simulink model "f8_VPP_demo_DER2"  (R2019b)
settings: Solver=VariableStepAuto  StartTime=0.0  StopTime=2  RelTol=1e-3
PreLoadFcn:
  | sr=0;ss=1;
InitFcn:
  | sr=0;ss=1;
undefined symbols (not defined in the file): Ion, Lithium
libraries: powerlib x185, powerlib_meascontrol x45, electricdrivelib x3, re_lib x3
(part 2 of 2)

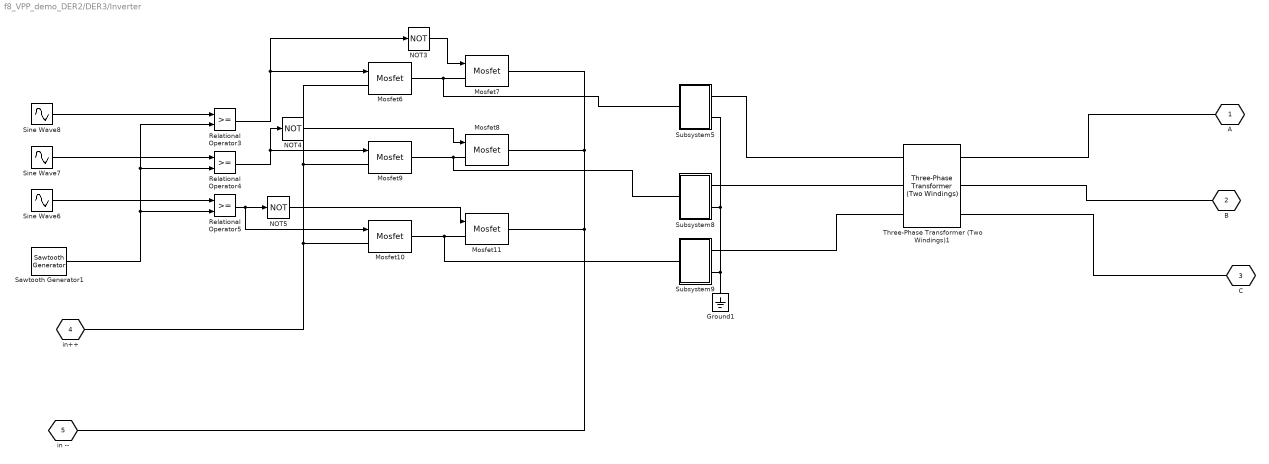
== system f8_VPP_demo_DER2/DER3/Inverter ==
  Ground1 : powerlib/Elements/Ground  LConnTagsString=a
      settings: SourceProductName=Simscape Electrical
  Mosfet{6..11} (6 alike) : powerlib/Power Electronics/Mosfet  Ron=0.1  Lon=0  Rd=0.01  Vfd=0  IC=0  Rs=1e5  Cs=inf  Measurements=off
      settings: SourceProductName=Simscape Electrical
  NOT3 : Logic  Operator=NOT  IconShape=distinctive  AllPortsSameDT=off  OutDataTypeStr=boolean
  NOT4 : Logic  Operator=NOT  IconShape=distinctive  AllPortsSameDT=off  OutDataTypeStr=boolean
  NOT5 : Logic  Operator=NOT  IconShape=distinctive  AllPortsSameDT=off  OutDataTypeStr=boolean
  Relational Operator3 : RelationalOperator  OutDataTypeStr=boolean  ZeroCross=off  RndMeth=Simplest
  Relational Operator4 : RelationalOperator  OutDataTypeStr=boolean  ZeroCross=off  RndMeth=Simplest
  Relational Operator5 : RelationalOperator  OutDataTypeStr=boolean  ZeroCross=off  RndMeth=Simplest
  Sawtooth Generator1 : powerlib_meascontrol/Pulse & Signal Generators/Sawtooth Generator  Freq=1e3  Phase=180  Ts=0
      settings: SourceProductName=Simscape Electrical
  Sine Wave6 : Sin  Frequency=2*pi*50  Phase=4*pi/3  SampleTime=0
  Sine Wave7 : Sin  Frequency=2*pi*50  Phase=2*pi/3  SampleTime=0
  Sine Wave8 : Sin  Frequency=2*pi*50  SampleTime=0
  Subsystem5 : Subsystem
  Subsystem8 : Subsystem
  Subsystem9 : Subsystem
  Three-Phase Transformer (Two Windings)1 : powerlib/Elements/Three-Phase Transformer (Two Windings)  Winding1Connection=Yg  Winding2Connection=Yg  CoreType=Three single-phase transformers  SetSaturation=off  Hysteresis=off  DataFile='hysteresis'  SetInitialFlux=off  Measurements=None  UNITS=pu  NominalPower=[ 1e3 , 50 ]  Winding1=[ 31.5 , 0.002 , 0.08 ]  Winding2=[ 240 , 0.002 , 0.08 ]  Rm=500  Lm=500  L0=0.5  Saturation=[ 0,0 ; 0.0024,1.2 ; 1.0,1.52 ]  InitialFluxes=[ 0.8 , -0.8 , 0.7 ]  BreakLoop=off  DiscreteSolver=Trapezoidal iterative  DataType=off  TransfoNumber=1
      settings: SourceProductName=Simscape Electrical
  A : PMIOPort  Tag=PMCPort  Side=Right
  B : PMIOPort  Tag=PMCPort  Port=2  Side=Right
  C : PMIOPort  Tag=PMCPort  Port=3  Side=Right
  in++ : PMIOPort  Tag=PMCPort  Port=4  Side=Left
  in -- : PMIOPort  Tag=PMCPort  Port=5  Side=Left
  wires:
  NOT5/1 -> Mosfet11/1
  Sine Wave6/1 -> Relational Operator5/1
  Sine Wave7/1 -> Relational Operator4/1
  Relational Operator4/1 -> Mosfet9/1, NOT4/1
  NOT4/1 -> Mosfet8/1
  Sawtooth Generator1/1 -> Relational Operator3/2, Relational Operator4/2, Relational Operator5/2
  Sine Wave8/1 -> Relational Operator3/1
  NOT3/1 -> Mosfet7/1
  Relational Operator5/1 -> Mosfet10/1, NOT5/1
  Relational Operator3/1 -> NOT3/1, Mosfet6/1
  connections:
  Mosfet10/LConn1 -- in++/RConn1 -- Mosfet9/LConn1 -- Mosfet6/LConn1
  Three-Phase Transformer (Two Windings)1/LConn3 -- Subsystem9/RConn1
  Mosfet9/RConn1 -- Mosfet8/LConn1 -- Subsystem8/LConn1
  Subsystem8/RConn1 -- Three-Phase Transformer (Two Windings)1/LConn2
  Mosfet11/LConn1 -- Mosfet10/RConn1 -- Subsystem9/LConn1
  Three-Phase Transformer (Two Windings)1/LConn1 -- Subsystem5/RConn1
  Mosfet6/RConn1 -- Mosfet7/LConn1 -- Subsystem5/LConn1
  Mosfet7/RConn1 -- Mosfet8/RConn1 -- in --/RConn1 -- Mosfet11/RConn1
  Subsystem9/RConn2 -- Ground1/LConn1 -- Subsystem8/RConn2 -- Subsystem5/RConn2
  Three-Phase Transformer (Two Windings)1/RConn3 -- C/RConn1
  Three-Phase Transformer (Two Windings)1/RConn2 -- B/RConn1
  Three-Phase Transformer (Two Windings)1/RConn1 -- A/RConn1

== system f8_VPP_demo_DER2/DER3/breaker_3phase1 ==
  c_breaker : Inport
  Breaker : powerlib/Elements/Breaker  InitialState=0  SwitchingTimes="[1/60  5/60]"  External=on  BreakerResistance=0.01  SnubberResistance=1e6  SnubberCapacitance=inf  Measurements=None  MoreParameters=on  NoBreakLoop=off
      settings: SourceProductName=Simscape Electrical
  Breaker1 : powerlib/Elements/Breaker  InitialState=0  SwitchingTimes="[1/60  5/60]"  External=on  BreakerResistance=0.01  SnubberResistance=1e6  SnubberCapacitance=inf  Measurements=None  MoreParameters=on  NoBreakLoop=off
      settings: SourceProductName=Simscape Electrical
  Breaker2 : powerlib/Elements/Breaker  InitialState=0  SwitchingTimes="[1/60  5/60]"  External=on  BreakerResistance=0.01  SnubberResistance=1e6  SnubberCapacitance=inf  Measurements=None  MoreParameters=on  NoBreakLoop=off
      settings: SourceProductName=Simscape Electrical
  a : PMIOPort  Tag=PMCPort  Side=Right
  A : PMIOPort  Tag=PMCPort  Port=2  Side=Left
  B : PMIOPort  Tag=PMCPort  Port=3  Side=Left
  C : PMIOPort  Tag=PMCPort  Port=4  Side=Left
  b : PMIOPort  Tag=PMCPort  Port=5  Side=Right
  c : PMIOPort  Tag=PMCPort  Port=6  Side=Right
  wires:
  c_breaker/1 -> Breaker1/1, Breaker2/1, Breaker/1
  connections:
  B/RConn1 -- Breaker1/LConn1
  A/RConn1 -- Breaker/LConn1
  c/RConn1 -- Breaker2/RConn1
  a/RConn1 -- Breaker/RConn1
  b/RConn1 -- Breaker1/RConn1
  C/RConn1 -- Breaker2/LConn1

== system f8_VPP_demo_DER2/DER3/power Measurement ==
  Current Measurement1 : powerlib/Measurements/Current Measurement  PhasorSimulation=off  OutputType=Complex  PSBequivalent=0
      settings: SourceProductName=Simscape Electrical
  First-Order Filter : powerlib_meascontrol/Filters/First-Order Filter  FilterType=Lowpass  Tc=100e-3  Ts=0  Initialize=off  Vac_Init=[0, 0, 50]  Vdc_Init=0  PlotResponse=off  FreqRange="[0,  200,  1]"
      settings: SourceProductName=Simscape Electrical
  First-Order Filter1 : powerlib_meascontrol/Filters/First-Order Filter  FilterType=Lowpass  Tc=100e-3  Ts=0  Initialize=off  Vac_Init=[0, 0, 50]  Vdc_Init=0  PlotResponse=off  FreqRange="[0,  200,  1]"
      settings: SourceProductName=Simscape Electrical
  Gain : Gain  Gain=3
  Ground1 : powerlib/Elements/Ground  LConnTagsString=a
      settings: SourceProductName=Simscape Electrical
  Product : Product
  RMS : powerlib_meascontrol/Measurements/RMS  TrueRMS=on  Freq=50  RMSInit=210  Ts=0.001
      settings: SourceProductName=Simscape Electrical
  RMS1 : powerlib_meascontrol/Measurements/RMS  TrueRMS=on  Freq=50  RMSInit=210  Ts=0.001
      settings: SourceProductName=Simscape Electrical
  Scope{,1..3} (4 alike) : Scope
  Voltage Measurement1 : powerlib/Measurements/Voltage Measurement  PhasorSimulation=off  OutputType=Complex  PSBequivalent=0
      settings: SourceProductName=Simscape Electrical
  "out " : PMIOPort  Tag=PMCPort  Side=Right
  in : PMIOPort  Tag=PMCPort  Port=2  Side=Left
  m : Outport
  wires:
  Current Measurement1/1 -> Scope1/1, RMS1/1
  Gain/1 -> m/1
  RMS/1 -> First-Order Filter/1
  RMS1/1 -> First-Order Filter1/1
  Voltage Measurement1/1 -> Scope/1, RMS/1
  First-Order Filter1/1 -> Product/1, Scope2/1
  First-Order Filter/1 -> Scope3/1, Product/2
  Product/1 -> Gain/1
  connections:
  Ground1/LConn1 -- Voltage Measurement1/LConn2
  Current Measurement1/LConn1 -- in/RConn1 -- Voltage Measurement1/LConn1
  "out "/RConn1 -- Current Measurement1/RConn1

== system f8_VPP_demo_DER2/DER3/solar system  ==
  Temp : Inport
  Irr : Inport  Port=2
  Bus Selector : BusSelector  OutputSignals=V_PV
  Current Measurement1 : powerlib/Measurements/Current Measurement  PhasorSimulation=off  OutputType=Complex  PSBequivalent=0
  PV Array : re_lib/Solar/PV Array  Npar=40  Nser=10  PlotType=array @ 1000 W/m2 & specified temperatures  S_vec="[ 1000  500  100 ]"  Temp_C_vec="[ 45 25  ]"  ModuleName=1Soltech 1STH-215-P  PlotWhenSelected=off  Pm=213.15  Ncell=60  Voc=36.3  Isc=7.84  Vm=29  Im=7.35  beta_Voc_pc=-0.36099  alpha_Isc_pc=0.102  beta_Voc=-0.13104  alpha_Isc=0.007997  IL=7.8649  I0=2.9259e-10  nI=0.98117  Rsh=313.3991  Rs=0.39383  BAL=off  Tc=1e-6  Tfilter=5e-5
      settings: SourceProductName=Simscape Electrical
  Scope2 : Scope
  Scope3 : Scope
  Series RLC Branch1 : powerlib/Elements/Series RLC Branch  LConnTagsString=__new0  RConnTagsString=__new0  BranchType=R  Resistance=1000000  Inductance=1e-3  SetiL0=off  InitialCurrent=0  Capacitance=1e-6  Setx0=off  InitialVoltage=0  Measurements=None
      settings: SourceProductName=Simscape Electrical
  baterry ++ : PMIOPort  Tag=PMCPort  Side=Right
  baterry -- : PMIOPort  Tag=PMCPort  Port=2  Side=Right
  wires:
  Current Measurement1/1 -> Scope3/1
  Temp/1 -> PV Array/2
  Irr/1 -> PV Array/1
  PV Array/1 -> Bus Selector/1
  Bus Selector/1 -> Scope2/1  "<V_PV>"
  connections:
  PV Array/RConn2 -- baterry --/RConn1 -- Series RLC Branch1/RConn1
  Current Measurement1/RConn1 -- baterry ++/RConn1
  PV Array/RConn1 -- Current Measurement1/LConn1 -- Series RLC Branch1/LConn1

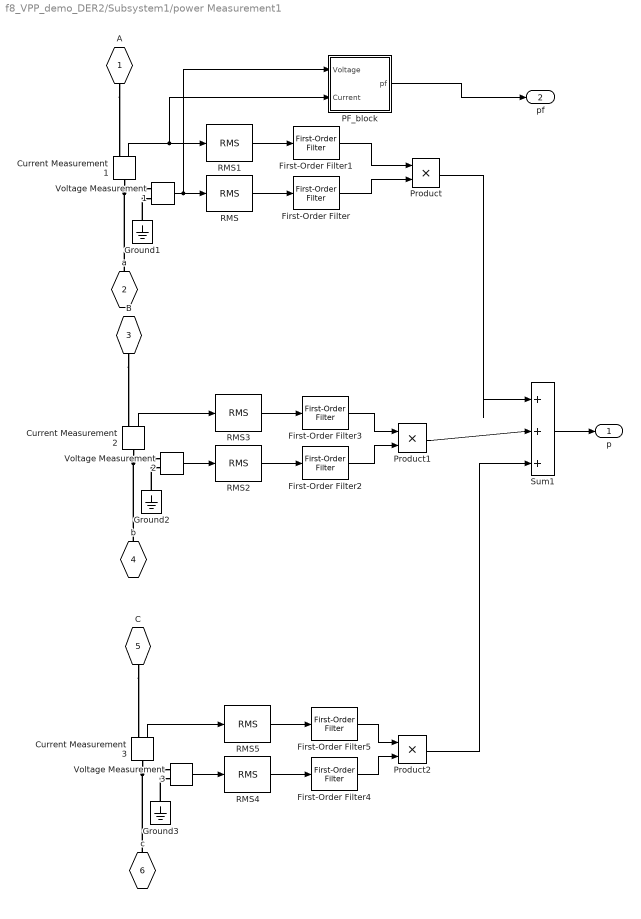
== system f8_VPP_demo_DER2/Subsystem1/power Measurement1 ==
  Current Measurement1 : powerlib/Measurements/Current Measurement  PhasorSimulation=off  OutputType=Complex  PSBequivalent=0
      settings: SourceProductName=Simscape Electrical
  Current Measurement2 : powerlib/Measurements/Current Measurement  PhasorSimulation=off  OutputType=Complex  PSBequivalent=0
      settings: SourceProductName=Simscape Electrical
  Current Measurement3 : powerlib/Measurements/Current Measurement  PhasorSimulation=off  OutputType=Complex  PSBequivalent=0
      settings: SourceProductName=Simscape Electrical
  First-Order Filter{,1..5} (6 alike) : powerlib_meascontrol/Filters/First-Order Filter  FilterType=Lowpass  Tc=100e-3  Ts=0  Initialize=off  Vac_Init=[0, 0, 50]  Vdc_Init=0  PlotResponse=off  FreqRange="[0,  200,  1]"
      settings: SourceProductName=Simscape Electrical
  Ground1 : powerlib/Elements/Ground  LConnTagsString=a
      settings: SourceProductName=Simscape Electrical
  Ground2 : powerlib/Elements/Ground  LConnTagsString=a
      settings: SourceProductName=Simscape Electrical
  Ground3 : powerlib/Elements/Ground  LConnTagsString=a
      settings: SourceProductName=Simscape Electrical
  PF_block : Subsystem
  Product : Product
  Product1 : Product
  Product2 : Product
  RMS{,1..5} (6 alike) : powerlib_meascontrol/Measurements/RMS  TrueRMS=on  Freq=50  RMSInit=210  Ts=0.001
      settings: SourceProductName=Simscape Electrical
  Sum1 : Sum  Inputs=|+++
  Voltage Measurement1 : powerlib/Measurements/Voltage Measurement  PhasorSimulation=off  OutputType=Complex  PSBequivalent=0
      settings: SourceProductName=Simscape Electrical
  Voltage Measurement2 : powerlib/Measurements/Voltage Measurement  PhasorSimulation=off  OutputType=Complex  PSBequivalent=0
      settings: SourceProductName=Simscape Electrical
  Voltage Measurement3 : powerlib/Measurements/Voltage Measurement  PhasorSimulation=off  OutputType=Complex  PSBequivalent=0
      settings: SourceProductName=Simscape Electrical
  "A " : PMIOPort  Tag=PMCPort  Side=Right
  a : PMIOPort  Tag=PMCPort  Port=2  Side=Left
  B : PMIOPort  Tag=PMCPort  Port=3  Side=Right
  b : PMIOPort  Tag=PMCPort  Port=4  Side=Left
  C : PMIOPort  Tag=PMCPort  Port=5  Side=Right
  c : PMIOPort  Tag=PMCPort  Port=6  Side=Left
  p : Outport
  pf : Outport  Port=2
  wires:
  Current Measurement1/1 -> PF_block/2(Current), RMS1/1
  Sum1/1 -> p/1
  RMS/1 -> First-Order Filter/1
  RMS1/1 -> First-Order Filter1/1
  Voltage Measurement1/1 -> PF_block/1(Voltage), RMS/1
  First-Order Filter1/1 -> Product/1
  First-Order Filter/1 -> Product/2
  Product/1 -> Sum1/1
  Voltage Measurement2/1 -> RMS2/1
  RMS3/1 -> First-Order Filter3/1
  RMS2/1 -> First-Order Filter2/1
  Current Measurement2/1 -> RMS3/1
  Current Measurement3/1 -> RMS5/1
  RMS4/1 -> First-Order Filter4/1
  RMS5/1 -> First-Order Filter5/1
  Voltage Measurement3/1 -> RMS4/1
  First-Order Filter3/1 -> Product1/1
  First-Order Filter2/1 -> Product1/2
  First-Order Filter5/1 -> Product2/1
  First-Order Filter4/1 -> Product2/2
  Product1/1 -> Sum1/2
  Product2/1 -> Sum1/3
  PF_block/1(pf) -> pf/1
  connections:
  Ground1/LConn1 -- Voltage Measurement1/LConn2
  Current Measurement1/LConn1 -- a/RConn1 -- Voltage Measurement1/LConn1
  "A "/RConn1 -- Current Measurement1/RConn1
  b/RConn1 -- Current Measurement2/LConn1 -- Voltage Measurement2/LConn1
  B/RConn1 -- Current Measurement2/RConn1
  Ground2/LConn1 -- Voltage Measurement2/LConn2
  c/RConn1 -- Voltage Measurement3/LConn1 -- Current Measurement3/LConn1
  Ground3/LConn1 -- Voltage Measurement3/LConn2
  C/RConn1 -- Current Measurement3/RConn1

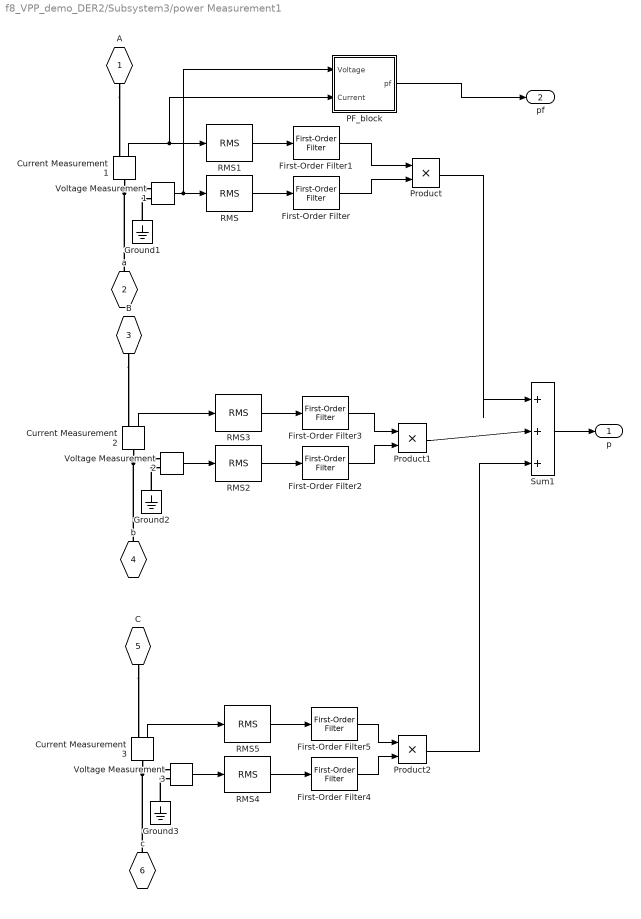
== system f8_VPP_demo_DER2/Subsystem3/power Measurement1 ==
  Current Measurement1 : powerlib/Measurements/Current Measurement  PhasorSimulation=off  OutputType=Complex  PSBequivalent=0
      settings: SourceProductName=Simscape Electrical
  Current Measurement2 : powerlib/Measurements/Current Measurement  PhasorSimulation=off  OutputType=Complex  PSBequivalent=0
      settings: SourceProductName=Simscape Electrical
  Current Measurement3 : powerlib/Measurements/Current Measurement  PhasorSimulation=off  OutputType=Complex  PSBequivalent=0
      settings: SourceProductName=Simscape Electrical
  First-Order Filter{,1..5} (6 alike) : powerlib_meascontrol/Filters/First-Order Filter  FilterType=Lowpass  Tc=100e-3  Ts=0  Initialize=off  Vac_Init=[0, 0, 50]  Vdc_Init=0  PlotResponse=off  FreqRange="[0,  200,  1]"
      settings: SourceProductName=Simscape Electrical
  Ground1 : powerlib/Elements/Ground  LConnTagsString=a
      settings: SourceProductName=Simscape Electrical
  Ground2 : powerlib/Elements/Ground  LConnTagsString=a
      settings: SourceProductName=Simscape Electrical
  Ground3 : powerlib/Elements/Ground  LConnTagsString=a
      settings: SourceProductName=Simscape Electrical
  PF_block : Subsystem
  Product : Product
  Product1 : Product
  Product2 : Product
  RMS{,1..5} (6 alike) : powerlib_meascontrol/Measurements/RMS  TrueRMS=on  Freq=50  RMSInit=210  Ts=0.001
      settings: SourceProductName=Simscape Electrical
  Sum1 : Sum  Inputs=|+++
  Voltage Measurement1 : powerlib/Measurements/Voltage Measurement  PhasorSimulation=off  OutputType=Complex  PSBequivalent=0
      settings: SourceProductName=Simscape Electrical
  Voltage Measurement2 : powerlib/Measurements/Voltage Measurement  PhasorSimulation=off  OutputType=Complex  PSBequivalent=0
      settings: SourceProductName=Simscape Electrical
  Voltage Measurement3 : powerlib/Measurements/Voltage Measurement  PhasorSimulation=off  OutputType=Complex  PSBequivalent=0
      settings: SourceProductName=Simscape Electrical
  "A " : PMIOPort  Tag=PMCPort  Side=Right
  a : PMIOPort  Tag=PMCPort  Port=2  Side=Left
  B : PMIOPort  Tag=PMCPort  Port=3  Side=Right
  b : PMIOPort  Tag=PMCPort  Port=4  Side=Left
  C : PMIOPort  Tag=PMCPort  Port=5  Side=Right
  c : PMIOPort  Tag=PMCPort  Port=6  Side=Left
  p : Outport
  pf : Outport  Port=2
  wires:
  Current Measurement1/1 -> PF_block/2(Current), RMS1/1
  Sum1/1 -> p/1
  RMS/1 -> First-Order Filter/1
  RMS1/1 -> First-Order Filter1/1
  Voltage Measurement1/1 -> PF_block/1(Voltage), RMS/1
  First-Order Filter1/1 -> Product/1
  First-Order Filter/1 -> Product/2
  Product/1 -> Sum1/1
  Voltage Measurement2/1 -> RMS2/1
  RMS3/1 -> First-Order Filter3/1
  RMS2/1 -> First-Order Filter2/1
  Current Measurement2/1 -> RMS3/1
  Current Measurement3/1 -> RMS5/1
  RMS4/1 -> First-Order Filter4/1
  RMS5/1 -> First-Order Filter5/1
  Voltage Measurement3/1 -> RMS4/1
  First-Order Filter3/1 -> Product1/1
  First-Order Filter2/1 -> Product1/2
  First-Order Filter5/1 -> Product2/1
  First-Order Filter4/1 -> Product2/2
  Product1/1 -> Sum1/2
  Product2/1 -> Sum1/3
  PF_block/1(pf) -> pf/1
  connections:
  Ground1/LConn1 -- Voltage Measurement1/LConn2
  Current Measurement1/LConn1 -- a/RConn1 -- Voltage Measurement1/LConn1
  "A "/RConn1 -- Current Measurement1/RConn1
  b/RConn1 -- Current Measurement2/LConn1 -- Voltage Measurement2/LConn1
  B/RConn1 -- Current Measurement2/RConn1
  Ground2/LConn1 -- Voltage Measurement2/LConn2
  c/RConn1 -- Voltage Measurement3/LConn1 -- Current Measurement3/LConn1
  Ground3/LConn1 -- Voltage Measurement3/LConn2
  C/RConn1 -- Current Measurement3/RConn1

== system f8_VPP_demo_DER2/DER1/Inverter/Subsystem5 ==
  Series RLC Branch{,2,5..6} (4 alike) : powerlib/Elements/Series RLC Branch  LConnTagsString=__new0  RConnTagsString=__new0  BranchType=L  Resistance=1  Inductance=92e-3  SetiL0=off  InitialCurrent=0  Capacitance=1e-6  Setx0=off  InitialVoltage=0  Measurements=None
      settings: SourceProductName=Simscape Electrical
  Series RLC Branch1 : powerlib/Elements/Series RLC Branch  LConnTagsString=__new0  RConnTagsString=__new0  BranchType=C  Resistance=1  Inductance=1e-3  SetiL0=off  InitialCurrent=0  Capacitance=110e-6  Setx0=off  InitialVoltage=0  Measurements=None
      settings: SourceProductName=Simscape Electrical
  Series RLC Branch11 : powerlib/Elements/Series RLC Branch  LConnTagsString=__new0  RConnTagsString=__new0  BranchType=R  Resistance=1  Inductance=1e-3  SetiL0=off  InitialCurrent=0  Capacitance=110e-6  Setx0=off  InitialVoltage=0  Measurements=None
      settings: SourceProductName=Simscape Electrical
  Series RLC Branch3 : powerlib/Elements/Series RLC Branch  LConnTagsString=__new0  RConnTagsString=__new0  BranchType=R  Resistance=500  Inductance=1e-3  SetiL0=off  InitialCurrent=0  Capacitance=110e-6  Setx0=off  InitialVoltage=0  Measurements=None
      settings: SourceProductName=Simscape Electrical
  Series RLC Branch4 : powerlib/Elements/Series RLC Branch  LConnTagsString=__new0  RConnTagsString=__new0  BranchType=R  Resistance=10  Inductance=1e-3  SetiL0=off  InitialCurrent=0  Capacitance=110e-6  Setx0=off  InitialVoltage=0  Measurements=None
      settings: SourceProductName=Simscape Electrical
  Series RLC Branch7 : powerlib/Elements/Series RLC Branch  LConnTagsString=__new0  RConnTagsString=__new0  BranchType=C  Resistance=1  Inductance=1e-3  SetiL0=off  InitialCurrent=0  Capacitance=110e-6  Setx0=off  InitialVoltage=0  Measurements=None
      settings: SourceProductName=Simscape Electrical
  Connection Port : PMIOPort  Tag=PMCPort  Side=Left
  Connection Port1 : PMIOPort  Tag=PMCPort  Port=2  Side=Right
  Connection Port3 : PMIOPort  Tag=PMCPort  Port=3  Side=Right
  connections:
  Connection Port/RConn1 -- Series RLC Branch/LConn1
  Series RLC Branch/RConn1 -- Series RLC Branch2/LConn1 -- Series RLC Branch1/RConn1
  Series RLC Branch5/LConn1 -- Series RLC Branch11/RConn1 -- Series RLC Branch7/LConn1
  Series RLC Branch5/RConn1 -- Series RLC Branch6/RConn1 -- Series RLC Branch4/LConn1 -- Connection Port3/RConn1 -- Series RLC Branch3/LConn1 -- Series RLC Branch1/LConn1
  Series RLC Branch3/RConn1 -- Series RLC Branch11/LConn1 -- Series RLC Branch2/RConn1
  Series RLC Branch6/LConn1 -- Series RLC Branch4/RConn1 -- Connection Port1/RConn1 -- Series RLC Branch7/RConn1

== system f8_VPP_demo_DER2/DER1/Inverter/Subsystem8 ==
  Series RLC Branch{,2,5..6} (4 alike) : powerlib/Elements/Series RLC Branch  LConnTagsString=__new0  RConnTagsString=__new0  BranchType=L  Resistance=1  Inductance=92e-3  SetiL0=off  InitialCurrent=0  Capacitance=1e-6  Setx0=off  InitialVoltage=0  Measurements=None
      settings: SourceProductName=Simscape Electrical
  Series RLC Branch1 : powerlib/Elements/Series RLC Branch  LConnTagsString=__new0  RConnTagsString=__new0  BranchType=C  Resistance=1  Inductance=1e-3  SetiL0=off  InitialCurrent=0  Capacitance=110e-6  Setx0=off  InitialVoltage=0  Measurements=None
      settings: SourceProductName=Simscape Electrical
  Series RLC Branch11 : powerlib/Elements/Series RLC Branch  LConnTagsString=__new0  RConnTagsString=__new0  BranchType=R  Resistance=1  Inductance=1e-3  SetiL0=off  InitialCurrent=0  Capacitance=110e-6  Setx0=off  InitialVoltage=0  Measurements=None
      settings: SourceProductName=Simscape Electrical
  Series RLC Branch3 : powerlib/Elements/Series RLC Branch  LConnTagsString=__new0  RConnTagsString=__new0  BranchType=R  Resistance=500  Inductance=1e-3  SetiL0=off  InitialCurrent=0  Capacitance=110e-6  Setx0=off  InitialVoltage=0  Measurements=None
      settings: SourceProductName=Simscape Electrical
  Series RLC Branch4 : powerlib/Elements/Series RLC Branch  LConnTagsString=__new0  RConnTagsString=__new0  BranchType=R  Resistance=10  Inductance=1e-3  SetiL0=off  InitialCurrent=0  Capacitance=110e-6  Setx0=off  InitialVoltage=0  Measurements=None
      settings: SourceProductName=Simscape Electrical
  Series RLC Branch7 : powerlib/Elements/Series RLC Branch  LConnTagsString=__new0  RConnTagsString=__new0  BranchType=C  Resistance=1  Inductance=1e-3  SetiL0=off  InitialCurrent=0  Capacitance=110e-6  Setx0=off  InitialVoltage=0  Measurements=None
      settings: SourceProductName=Simscape Electrical
  Connection Port : PMIOPort  Tag=PMCPort  Side=Left
  Connection Port1 : PMIOPort  Tag=PMCPort  Port=2  Side=Right
  Connection Port3 : PMIOPort  Tag=PMCPort  Port=3  Side=Right
  connections:
  Series RLC Branch7/RConn1 -- Series RLC Branch6/LConn1 -- Series RLC Branch4/RConn1 -- Connection Port1/RConn1
  Series RLC Branch3/RConn1 -- Series RLC Branch2/RConn1 -- Series RLC Branch11/LConn1
  Series RLC Branch6/RConn1 -- Series RLC Branch3/LConn1 -- Series RLC Branch1/LConn1 -- Series RLC Branch5/RConn1 -- Series RLC Branch4/LConn1 -- Connection Port3/RConn1
  Series RLC Branch5/LConn1 -- Series RLC Branch7/LConn1 -- Series RLC Branch11/RConn1
  Series RLC Branch1/RConn1 -- Series RLC Branch2/LConn1 -- Series RLC Branch/RConn1
  Connection Port/RConn1 -- Series RLC Branch/LConn1

== system f8_VPP_demo_DER2/DER1/Inverter/Subsystem9 ==
  Series RLC Branch{,2,5..6} (4 alike) : powerlib/Elements/Series RLC Branch  LConnTagsString=__new0  RConnTagsString=__new0  BranchType=L  Resistance=1  Inductance=92e-3  SetiL0=off  InitialCurrent=0  Capacitance=1e-6  Setx0=off  InitialVoltage=0  Measurements=None
      settings: SourceProductName=Simscape Electrical
  Series RLC Branch1 : powerlib/Elements/Series RLC Branch  LConnTagsString=__new0  RConnTagsString=__new0  BranchType=C  Resistance=1  Inductance=1e-3  SetiL0=off  InitialCurrent=0  Capacitance=110e-6  Setx0=off  InitialVoltage=0  Measurements=None
      settings: SourceProductName=Simscape Electrical
  Series RLC Branch11 : powerlib/Elements/Series RLC Branch  LConnTagsString=__new0  RConnTagsString=__new0  BranchType=R  Resistance=1  Inductance=1e-3  SetiL0=off  InitialCurrent=0  Capacitance=110e-6  Setx0=off  InitialVoltage=0  Measurements=None
      settings: SourceProductName=Simscape Electrical
  Series RLC Branch3 : powerlib/Elements/Series RLC Branch  LConnTagsString=__new0  RConnTagsString=__new0  BranchType=R  Resistance=500  Inductance=1e-3  SetiL0=off  InitialCurrent=0  Capacitance=110e-6  Setx0=off  InitialVoltage=0  Measurements=None
      settings: SourceProductName=Simscape Electrical
  Series RLC Branch4 : powerlib/Elements/Series RLC Branch  LConnTagsString=__new0  RConnTagsString=__new0  BranchType=R  Resistance=10  Inductance=1e-3  SetiL0=off  InitialCurrent=0  Capacitance=110e-6  Setx0=off  InitialVoltage=0  Measurements=None
      settings: SourceProductName=Simscape Electrical
  Series RLC Branch7 : powerlib/Elements/Series RLC Branch  LConnTagsString=__new0  RConnTagsString=__new0  BranchType=C  Resistance=1  Inductance=1e-3  SetiL0=off  InitialCurrent=0  Capacitance=110e-6  Setx0=off  InitialVoltage=0  Measurements=None
      settings: SourceProductName=Simscape Electrical
  Connection Port : PMIOPort  Tag=PMCPort  Side=Left
  Connection Port1 : PMIOPort  Tag=PMCPort  Port=2  Side=Right
  Connection Port3 : PMIOPort  Tag=PMCPort  Port=3  Side=Right
  connections:
  Connection Port/RConn1 -- Series RLC Branch/LConn1
  Series RLC Branch/RConn1 -- Series RLC Branch2/LConn1 -- Series RLC Branch1/RConn1
  Series RLC Branch11/RConn1 -- Series RLC Branch7/LConn1 -- Series RLC Branch5/LConn1
  Connection Port3/RConn1 -- Series RLC Branch4/LConn1 -- Series RLC Branch5/RConn1 -- Series RLC Branch3/LConn1 -- Series RLC Branch1/LConn1 -- Series RLC Branch6/RConn1
  Series RLC Branch11/LConn1 -- Series RLC Branch2/RConn1 -- Series RLC Branch3/RConn1
  Connection Port1/RConn1 -- Series RLC Branch4/RConn1 -- Series RLC Branch6/LConn1 -- Series RLC Branch7/RConn1

== system f8_VPP_demo_DER2/DER2/Inverter/Subsystem5 ==
  Series RLC Branch{,2,5..6} (4 alike) : powerlib/Elements/Series RLC Branch  LConnTagsString=__new0  RConnTagsString=__new0  BranchType=L  Resistance=1  Inductance=92e-3  SetiL0=off  InitialCurrent=0  Capacitance=1e-6  Setx0=off  InitialVoltage=0  Measurements=None
      settings: SourceProductName=Simscape Electrical
  Series RLC Branch1 : powerlib/Elements/Series RLC Branch  LConnTagsString=__new0  RConnTagsString=__new0  BranchType=C  Resistance=1  Inductance=1e-3  SetiL0=off  InitialCurrent=0  Capacitance=110e-6  Setx0=off  InitialVoltage=0  Measurements=None
      settings: SourceProductName=Simscape Electrical
  Series RLC Branch11 : powerlib/Elements/Series RLC Branch  LConnTagsString=__new0  RConnTagsString=__new0  BranchType=R  Resistance=1  Inductance=1e-3  SetiL0=off  InitialCurrent=0  Capacitance=110e-6  Setx0=off  InitialVoltage=0  Measurements=None
      settings: SourceProductName=Simscape Electrical
  Series RLC Branch3 : powerlib/Elements/Series RLC Branch  LConnTagsString=__new0  RConnTagsString=__new0  BranchType=R  Resistance=500  Inductance=1e-3  SetiL0=off  InitialCurrent=0  Capacitance=110e-6  Setx0=off  InitialVoltage=0  Measurements=None
      settings: SourceProductName=Simscape Electrical
  Series RLC Branch4 : powerlib/Elements/Series RLC Branch  LConnTagsString=__new0  RConnTagsString=__new0  BranchType=R  Resistance=10  Inductance=1e-3  SetiL0=off  InitialCurrent=0  Capacitance=110e-6  Setx0=off  InitialVoltage=0  Measurements=None
      settings: SourceProductName=Simscape Electrical
  Series RLC Branch7 : powerlib/Elements/Series RLC Branch  LConnTagsString=__new0  RConnTagsString=__new0  BranchType=C  Resistance=1  Inductance=1e-3  SetiL0=off  InitialCurrent=0  Capacitance=110e-6  Setx0=off  InitialVoltage=0  Measurements=None
      settings: SourceProductName=Simscape Electrical
  Connection Port : PMIOPort  Tag=PMCPort  Side=Left
  Connection Port1 : PMIOPort  Tag=PMCPort  Port=2  Side=Right
  Connection Port3 : PMIOPort  Tag=PMCPort  Port=3  Side=Right
  connections:
  Connection Port/RConn1 -- Series RLC Branch/LConn1
  Series RLC Branch/RConn1 -- Series RLC Branch2/LConn1 -- Series RLC Branch1/RConn1
  Series RLC Branch5/LConn1 -- Series RLC Branch11/RConn1 -- Series RLC Branch7/LConn1
  Series RLC Branch5/RConn1 -- Series RLC Branch6/RConn1 -- Series RLC Branch4/LConn1 -- Connection Port3/RConn1 -- Series RLC Branch3/LConn1 -- Series RLC Branch1/LConn1
  Series RLC Branch3/RConn1 -- Series RLC Branch11/LConn1 -- Series RLC Branch2/RConn1
  Series RLC Branch6/LConn1 -- Series RLC Branch4/RConn1 -- Connection Port1/RConn1 -- Series RLC Branch7/RConn1

== system f8_VPP_demo_DER2/DER2/Inverter/Subsystem8 ==
  Series RLC Branch{,2,5..6} (4 alike) : powerlib/Elements/Series RLC Branch  LConnTagsString=__new0  RConnTagsString=__new0  BranchType=L  Resistance=1  Inductance=92e-3  SetiL0=off  InitialCurrent=0  Capacitance=1e-6  Setx0=off  InitialVoltage=0  Measurements=None
      settings: SourceProductName=Simscape Electrical
  Series RLC Branch1 : powerlib/Elements/Series RLC Branch  LConnTagsString=__new0  RConnTagsString=__new0  BranchType=C  Resistance=1  Inductance=1e-3  SetiL0=off  InitialCurrent=0  Capacitance=110e-6  Setx0=off  InitialVoltage=0  Measurements=None
      settings: SourceProductName=Simscape Electrical
  Series RLC Branch11 : powerlib/Elements/Series RLC Branch  LConnTagsString=__new0  RConnTagsString=__new0  BranchType=R  Resistance=1  Inductance=1e-3  SetiL0=off  InitialCurrent=0  Capacitance=110e-6  Setx0=off  InitialVoltage=0  Measurements=None
      settings: SourceProductName=Simscape Electrical
  Series RLC Branch3 : powerlib/Elements/Series RLC Branch  LConnTagsString=__new0  RConnTagsString=__new0  BranchType=R  Resistance=500  Inductance=1e-3  SetiL0=off  InitialCurrent=0  Capacitance=110e-6  Setx0=off  InitialVoltage=0  Measurements=None
      settings: SourceProductName=Simscape Electrical
  Series RLC Branch4 : powerlib/Elements/Series RLC Branch  LConnTagsString=__new0  RConnTagsString=__new0  BranchType=R  Resistance=10  Inductance=1e-3  SetiL0=off  InitialCurrent=0  Capacitance=110e-6  Setx0=off  InitialVoltage=0  Measurements=None
      settings: SourceProductName=Simscape Electrical
  Series RLC Branch7 : powerlib/Elements/Series RLC Branch  LConnTagsString=__new0  RConnTagsString=__new0  BranchType=C  Resistance=1  Inductance=1e-3  SetiL0=off  InitialCurrent=0  Capacitance=110e-6  Setx0=off  InitialVoltage=0  Measurements=None
      settings: SourceProductName=Simscape Electrical
  Connection Port : PMIOPort  Tag=PMCPort  Side=Left
  Connection Port1 : PMIOPort  Tag=PMCPort  Port=2  Side=Right
  Connection Port3 : PMIOPort  Tag=PMCPort  Port=3  Side=Right
  connections:
  Series RLC Branch7/RConn1 -- Series RLC Branch6/LConn1 -- Series RLC Branch4/RConn1 -- Connection Port1/RConn1
  Series RLC Branch3/RConn1 -- Series RLC Branch2/RConn1 -- Series RLC Branch11/LConn1
  Series RLC Branch6/RConn1 -- Series RLC Branch3/LConn1 -- Series RLC Branch1/LConn1 -- Series RLC Branch5/RConn1 -- Series RLC Branch4/LConn1 -- Connection Port3/RConn1
  Series RLC Branch5/LConn1 -- Series RLC Branch7/LConn1 -- Series RLC Branch11/RConn1
  Series RLC Branch1/RConn1 -- Series RLC Branch2/LConn1 -- Series RLC Branch/RConn1
  Connection Port/RConn1 -- Series RLC Branch/LConn1

== system f8_VPP_demo_DER2/DER2/Inverter/Subsystem9 ==
  Series RLC Branch{,2,5..6} (4 alike) : powerlib/Elements/Series RLC Branch  LConnTagsString=__new0  RConnTagsString=__new0  BranchType=L  Resistance=1  Inductance=92e-3  SetiL0=off  InitialCurrent=0  Capacitance=1e-6  Setx0=off  InitialVoltage=0  Measurements=None
      settings: SourceProductName=Simscape Electrical
  Series RLC Branch1 : powerlib/Elements/Series RLC Branch  LConnTagsString=__new0  RConnTagsString=__new0  BranchType=C  Resistance=1  Inductance=1e-3  SetiL0=off  InitialCurrent=0  Capacitance=110e-6  Setx0=off  InitialVoltage=0  Measurements=None
      settings: SourceProductName=Simscape Electrical
  Series RLC Branch11 : powerlib/Elements/Series RLC Branch  LConnTagsString=__new0  RConnTagsString=__new0  BranchType=R  Resistance=1  Inductance=1e-3  SetiL0=off  InitialCurrent=0  Capacitance=110e-6  Setx0=off  InitialVoltage=0  Measurements=None
      settings: SourceProductName=Simscape Electrical
  Series RLC Branch3 : powerlib/Elements/Series RLC Branch  LConnTagsString=__new0  RConnTagsString=__new0  BranchType=R  Resistance=500  Inductance=1e-3  SetiL0=off  InitialCurrent=0  Capacitance=110e-6  Setx0=off  InitialVoltage=0  Measurements=None
      settings: SourceProductName=Simscape Electrical
  Series RLC Branch4 : powerlib/Elements/Series RLC Branch  LConnTagsString=__new0  RConnTagsString=__new0  BranchType=R  Resistance=10  Inductance=1e-3  SetiL0=off  InitialCurrent=0  Capacitance=110e-6  Setx0=off  InitialVoltage=0  Measurements=None
      settings: SourceProductName=Simscape Electrical
  Series RLC Branch7 : powerlib/Elements/Series RLC Branch  LConnTagsString=__new0  RConnTagsString=__new0  BranchType=C  Resistance=1  Inductance=1e-3  SetiL0=off  InitialCurrent=0  Capacitance=110e-6  Setx0=off  InitialVoltage=0  Measurements=None
      settings: SourceProductName=Simscape Electrical
  Connection Port : PMIOPort  Tag=PMCPort  Side=Left
  Connection Port1 : PMIOPort  Tag=PMCPort  Port=2  Side=Right
  Connection Port3 : PMIOPort  Tag=PMCPort  Port=3  Side=Right
  connections:
  Connection Port/RConn1 -- Series RLC Branch/LConn1
  Series RLC Branch/RConn1 -- Series RLC Branch2/LConn1 -- Series RLC Branch1/RConn1
  Series RLC Branch11/RConn1 -- Series RLC Branch7/LConn1 -- Series RLC Branch5/LConn1
  Connection Port3/RConn1 -- Series RLC Branch4/LConn1 -- Series RLC Branch5/RConn1 -- Series RLC Branch3/LConn1 -- Series RLC Branch1/LConn1 -- Series RLC Branch6/RConn1
  Series RLC Branch11/LConn1 -- Series RLC Branch2/RConn1 -- Series RLC Branch3/RConn1
  Connection Port1/RConn1 -- Series RLC Branch4/RConn1 -- Series RLC Branch6/LConn1 -- Series RLC Branch7/RConn1

== system f8_VPP_demo_DER2/DER3/Inverter/Subsystem5 ==
  Series RLC Branch{,2,5..6} (4 alike) : powerlib/Elements/Series RLC Branch  LConnTagsString=__new0  RConnTagsString=__new0  BranchType=L  Resistance=1  Inductance=92e-3  SetiL0=off  InitialCurrent=0  Capacitance=1e-6  Setx0=off  InitialVoltage=0  Measurements=None
      settings: SourceProductName=Simscape Electrical
  Series RLC Branch1 : powerlib/Elements/Series RLC Branch  LConnTagsString=__new0  RConnTagsString=__new0  BranchType=C  Resistance=1  Inductance=1e-3  SetiL0=off  InitialCurrent=0  Capacitance=110e-6  Setx0=off  InitialVoltage=0  Measurements=None
      settings: SourceProductName=Simscape Electrical
  Series RLC Branch11 : powerlib/Elements/Series RLC Branch  LConnTagsString=__new0  RConnTagsString=__new0  BranchType=R  Resistance=1  Inductance=1e-3  SetiL0=off  InitialCurrent=0  Capacitance=110e-6  Setx0=off  InitialVoltage=0  Measurements=None
      settings: SourceProductName=Simscape Electrical
  Series RLC Branch3 : powerlib/Elements/Series RLC Branch  LConnTagsString=__new0  RConnTagsString=__new0  BranchType=R  Resistance=500  Inductance=1e-3  SetiL0=off  InitialCurrent=0  Capacitance=110e-6  Setx0=off  InitialVoltage=0  Measurements=None
      settings: SourceProductName=Simscape Electrical
  Series RLC Branch4 : powerlib/Elements/Series RLC Branch  LConnTagsString=__new0  RConnTagsString=__new0  BranchType=R  Resistance=10  Inductance=1e-3  SetiL0=off  InitialCurrent=0  Capacitance=110e-6  Setx0=off  InitialVoltage=0  Measurements=None
      settings: SourceProductName=Simscape Electrical
  Series RLC Branch7 : powerlib/Elements/Series RLC Branch  LConnTagsString=__new0  RConnTagsString=__new0  BranchType=C  Resistance=1  Inductance=1e-3  SetiL0=off  InitialCurrent=0  Capacitance=110e-6  Setx0=off  InitialVoltage=0  Measurements=None
      settings: SourceProductName=Simscape Electrical
  Connection Port : PMIOPort  Tag=PMCPort  Side=Left
  Connection Port1 : PMIOPort  Tag=PMCPort  Port=2  Side=Right
  Connection Port3 : PMIOPort  Tag=PMCPort  Port=3  Side=Right
  connections:
  Connection Port/RConn1 -- Series RLC Branch/LConn1
  Series RLC Branch/RConn1 -- Series RLC Branch2/LConn1 -- Series RLC Branch1/RConn1
  Series RLC Branch5/LConn1 -- Series RLC Branch11/RConn1 -- Series RLC Branch7/LConn1
  Series RLC Branch5/RConn1 -- Series RLC Branch6/RConn1 -- Series RLC Branch4/LConn1 -- Connection Port3/RConn1 -- Series RLC Branch3/LConn1 -- Series RLC Branch1/LConn1
  Series RLC Branch3/RConn1 -- Series RLC Branch11/LConn1 -- Series RLC Branch2/RConn1
  Series RLC Branch6/LConn1 -- Series RLC Branch4/RConn1 -- Connection Port1/RConn1 -- Series RLC Branch7/RConn1

== system f8_VPP_demo_DER2/DER3/Inverter/Subsystem8 ==
  Series RLC Branch{,2,5..6} (4 alike) : powerlib/Elements/Series RLC Branch  LConnTagsString=__new0  RConnTagsString=__new0  BranchType=L  Resistance=1  Inductance=92e-3  SetiL0=off  InitialCurrent=0  Capacitance=1e-6  Setx0=off  InitialVoltage=0  Measurements=None
      settings: SourceProductName=Simscape Electrical
  Series RLC Branch1 : powerlib/Elements/Series RLC Branch  LConnTagsString=__new0  RConnTagsString=__new0  BranchType=C  Resistance=1  Inductance=1e-3  SetiL0=off  InitialCurrent=0  Capacitance=110e-6  Setx0=off  InitialVoltage=0  Measurements=None
      settings: SourceProductName=Simscape Electrical
  Series RLC Branch11 : powerlib/Elements/Series RLC Branch  LConnTagsString=__new0  RConnTagsString=__new0  BranchType=R  Resistance=1  Inductance=1e-3  SetiL0=off  InitialCurrent=0  Capacitance=110e-6  Setx0=off  InitialVoltage=0  Measurements=None
      settings: SourceProductName=Simscape Electrical
  Series RLC Branch3 : powerlib/Elements/Series RLC Branch  LConnTagsString=__new0  RConnTagsString=__new0  BranchType=R  Resistance=500  Inductance=1e-3  SetiL0=off  InitialCurrent=0  Capacitance=110e-6  Setx0=off  InitialVoltage=0  Measurements=None
      settings: SourceProductName=Simscape Electrical
  Series RLC Branch4 : powerlib/Elements/Series RLC Branch  LConnTagsString=__new0  RConnTagsString=__new0  BranchType=R  Resistance=10  Inductance=1e-3  SetiL0=off  InitialCurrent=0  Capacitance=110e-6  Setx0=off  InitialVoltage=0  Measurements=None
      settings: SourceProductName=Simscape Electrical
  Series RLC Branch7 : powerlib/Elements/Series RLC Branch  LConnTagsString=__new0  RConnTagsString=__new0  BranchType=C  Resistance=1  Inductance=1e-3  SetiL0=off  InitialCurrent=0  Capacitance=110e-6  Setx0=off  InitialVoltage=0  Measurements=None
      settings: SourceProductName=Simscape Electrical
  Connection Port : PMIOPort  Tag=PMCPort  Side=Left
  Connection Port1 : PMIOPort  Tag=PMCPort  Port=2  Side=Right
  Connection Port3 : PMIOPort  Tag=PMCPort  Port=3  Side=Right
  connections:
  Series RLC Branch7/RConn1 -- Series RLC Branch6/LConn1 -- Series RLC Branch4/RConn1 -- Connection Port1/RConn1
  Series RLC Branch3/RConn1 -- Series RLC Branch2/RConn1 -- Series RLC Branch11/LConn1
  Series RLC Branch6/RConn1 -- Series RLC Branch3/LConn1 -- Series RLC Branch1/LConn1 -- Series RLC Branch5/RConn1 -- Series RLC Branch4/LConn1 -- Connection Port3/RConn1
  Series RLC Branch5/LConn1 -- Series RLC Branch7/LConn1 -- Series RLC Branch11/RConn1
  Series RLC Branch1/RConn1 -- Series RLC Branch2/LConn1 -- Series RLC Branch/RConn1
  Connection Port/RConn1 -- Series RLC Branch/LConn1

== system f8_VPP_demo_DER2/DER3/Inverter/Subsystem9 ==
  Series RLC Branch{,2,5..6} (4 alike) : powerlib/Elements/Series RLC Branch  LConnTagsString=__new0  RConnTagsString=__new0  BranchType=L  Resistance=1  Inductance=92e-3  SetiL0=off  InitialCurrent=0  Capacitance=1e-6  Setx0=off  InitialVoltage=0  Measurements=None
      settings: SourceProductName=Simscape Electrical
  Series RLC Branch1 : powerlib/Elements/Series RLC Branch  LConnTagsString=__new0  RConnTagsString=__new0  BranchType=C  Resistance=1  Inductance=1e-3  SetiL0=off  InitialCurrent=0  Capacitance=110e-6  Setx0=off  InitialVoltage=0  Measurements=None
      settings: SourceProductName=Simscape Electrical
  Series RLC Branch11 : powerlib/Elements/Series RLC Branch  LConnTagsString=__new0  RConnTagsString=__new0  BranchType=R  Resistance=1  Inductance=1e-3  SetiL0=off  InitialCurrent=0  Capacitance=110e-6  Setx0=off  InitialVoltage=0  Measurements=None
      settings: SourceProductName=Simscape Electrical
  Series RLC Branch3 : powerlib/Elements/Series RLC Branch  LConnTagsString=__new0  RConnTagsString=__new0  BranchType=R  Resistance=500  Inductance=1e-3  SetiL0=off  InitialCurrent=0  Capacitance=110e-6  Setx0=off  InitialVoltage=0  Measurements=None
      settings: SourceProductName=Simscape Electrical
  Series RLC Branch4 : powerlib/Elements/Series RLC Branch  LConnTagsString=__new0  RConnTagsString=__new0  BranchType=R  Resistance=10  Inductance=1e-3  SetiL0=off  InitialCurrent=0  Capacitance=110e-6  Setx0=off  InitialVoltage=0  Measurements=None
      settings: SourceProductName=Simscape Electrical
  Series RLC Branch7 : powerlib/Elements/Series RLC Branch  LConnTagsString=__new0  RConnTagsString=__new0  BranchType=C  Resistance=1  Inductance=1e-3  SetiL0=off  InitialCurrent=0  Capacitance=110e-6  Setx0=off  InitialVoltage=0  Measurements=None
      settings: SourceProductName=Simscape Electrical
  Connection Port : PMIOPort  Tag=PMCPort  Side=Left
  Connection Port1 : PMIOPort  Tag=PMCPort  Port=2  Side=Right
  Connection Port3 : PMIOPort  Tag=PMCPort  Port=3  Side=Right
  connections:
  Connection Port/RConn1 -- Series RLC Branch/LConn1
  Series RLC Branch/RConn1 -- Series RLC Branch2/LConn1 -- Series RLC Branch1/RConn1
  Series RLC Branch11/RConn1 -- Series RLC Branch7/LConn1 -- Series RLC Branch5/LConn1
  Connection Port3/RConn1 -- Series RLC Branch4/LConn1 -- Series RLC Branch5/RConn1 -- Series RLC Branch3/LConn1 -- Series RLC Branch1/LConn1 -- Series RLC Branch6/RConn1
  Series RLC Branch11/LConn1 -- Series RLC Branch2/RConn1 -- Series RLC Branch3/RConn1
  Connection Port1/RConn1 -- Series RLC Branch4/RConn1 -- Series RLC Branch6/LConn1 -- Series RLC Branch7/RConn1

== system f8_VPP_demo_DER2/Subsystem1/power Measurement1/PF_block ==
  Voltage : Inport
  Current : Inport  Port=2
  A : Constant
  B : Constant
  First-Order Filter : powerlib_meascontrol/Filters/First-Order Filter  FilterType=Lowpass  Tc=100e-3  Ts=0  Initialize=off  Vac_Init=[0, 0, 50]  Vdc_Init=0  PlotResponse=off  FreqRange="[0,  200,  1]"
      settings: SourceProductName=Simscape Electrical
  G : Gain  Gain=2*pi*5
  M : Sum  Inputs=+-
  S1 : Integrator  ExternalReset=falling  ZeroCross=off
  S2 : Integrator  ExternalReset=falling  ZeroCross=off
  T : Trigonometry  Operator=cos
  pf : Outport
  wires:
  M/1 -> G/1
  Voltage/1 -> S1/2
  S2/1 -> M/2
  A/1 -> S1/1
  S1/1 -> M/1
  Current/1 -> S2/2
  G/1 -> T/1
  B/1 -> S2/1
  First-Order Filter/1 -> pf/1
  T/1 -> First-Order Filter/1

== system f8_VPP_demo_DER2/Subsystem3/power Measurement1/PF_block ==
  Voltage : Inport
  Current : Inport  Port=2
  A : Constant
  B : Constant
  First-Order Filter : powerlib_meascontrol/Filters/First-Order Filter  FilterType=Lowpass  Tc=100e-3  Ts=0  Initialize=off  Vac_Init=[0, 0, 50]  Vdc_Init=0  PlotResponse=off  FreqRange="[0,  200,  1]"
      settings: SourceProductName=Simscape Electrical
  G : Gain  Gain=2*pi*5
  M : Sum  Inputs=+-
  S1 : Integrator  ExternalReset=falling  ZeroCross=off
  S2 : Integrator  ExternalReset=falling  ZeroCross=off
  T : Trigonometry  Operator=cos
  pf : Outport
  wires:
  M/1 -> G/1
  Voltage/1 -> S1/2
  S2/1 -> M/2
  A/1 -> S1/1
  S1/1 -> M/1
  Current/1 -> S2/2
  G/1 -> T/1
  B/1 -> S2/1
  First-Order Filter/1 -> pf/1
  T/1 -> First-Order Filter/1

== matlab function f8_VPP_demo_DER2/Central control Router ==
  data: power input; powerPrev output; s1 input; s2 input; s3 input; powerPrev input; d1 input; d2 input; d3 input; d1 output; d2 output; d3 output
function [powerPrev,d1,d2,d3] = fcn(power,s1,s2,s3,powerPrev,d1,d2,d3)
    if (abs(powerPrev-power)>2000)
        powerPrev=power;
        discharge=[0 0 0];
        soc=[s1 s2 s3];
        while(power>25000)
            [m,i]=max(soc);
            soc(i)=0;
            if(m>10)
                discharge(i)=1;
                power=power-4000;
            end
        end
        d1=discharge(1);
        d2=discharge(2);
        d3=discharge(3);
    end
